simulink model "SmartHomeModelFinal"  (R2014a)
settings: Solver=ode45  StartTime=0.0  StopTime=inf  RelTol=1e-3
settings Model: Creator=Drazenko  LastModifiedBy=Drazenko

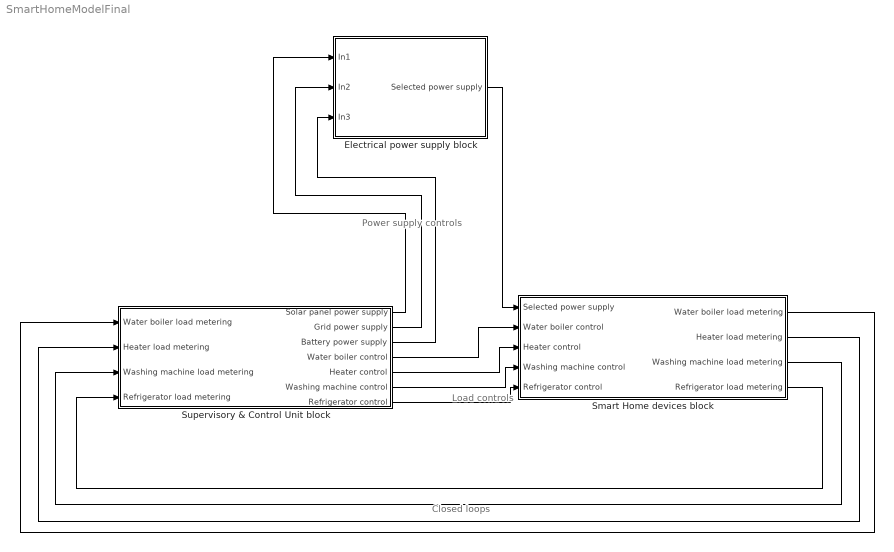
== system SmartHomeModelFinal ==
  note: Closed loops
  note: Load controls
  note: Power supply controls
  Electrical power supply block : Subsystem
  Smart Home devices block : Subsystem
  Supervisory & Control Unit block : Subsystem
  wires:
  Electrical power supply block/1(Selected power supply) -> Smart Home devices block/1(Selected power supply)
  Smart Home devices block/1(Water boiler load metering) -> Supervisory & Control Unit block/1(Water boiler load metering)
  Smart Home devices block/2(Heater load metering) -> Supervisory & Control Unit block/2(Heater load metering)
  Smart Home devices block/3(Washing machine load metering) -> Supervisory & Control Unit block/3(Washing machine load metering)
  Smart Home devices block/4(Refrigerator load metering) -> Supervisory & Control Unit block/4(Refrigerator load metering)
  Supervisory & Control Unit block/1(Solar panel power supply) -> Electrical power supply block/1(In1)
  Supervisory & Control Unit block/2(Grid power supply) -> Electrical power supply block/2(In2)
  Supervisory & Control Unit block/3(Battery power supply) -> Electrical power supply block/3(In3)
  Supervisory & Control Unit block/4(Water boiler control) -> Smart Home devices block/2(Water boiler control)
  Supervisory & Control Unit block/5(Heater control) -> Smart Home devices block/3(Heater control)
  Supervisory & Control Unit block/6(Washing machine control) -> Smart Home devices block/4(Washing machine control)
  Supervisory & Control Unit block/7(Refrigerator control) -> Smart Home devices block/5(Refrigerator control)

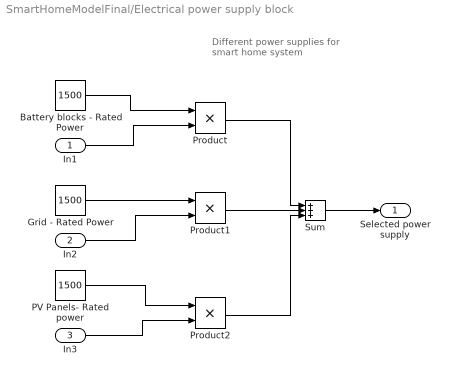
== system SmartHomeModelFinal/Electrical power supply block ==
  note: Different power supplies
      | for smart home system
  In1 : Inport
  In2 : Inport  Port=2
  In3 : Inport  Port=3
  Battery blocks - Rated Power : Constant  Value=1500
  Grid - Rated Power : Constant  Value=1500
  PV Panels- Rated power : Constant  Value=1500
  Product : Product
  Product1 : Product
  Product2 : Product
  Sum : Sum  Inputs=+++
  Selected power supply : Outport
  wires:
  Battery blocks - Rated Power/1 -> Product/1
  In1/1 -> Product/2
  Grid - Rated Power/1 -> Product1/1
  In2/1 -> Product1/2
  PV Panels- Rated power/1 -> Product2/1
  In3/1 -> Product2/2
  Product/1 -> Sum/1
  Product1/1 -> Sum/2
  Product2/1 -> Sum/3
  Sum/1 -> Selected power supply/1

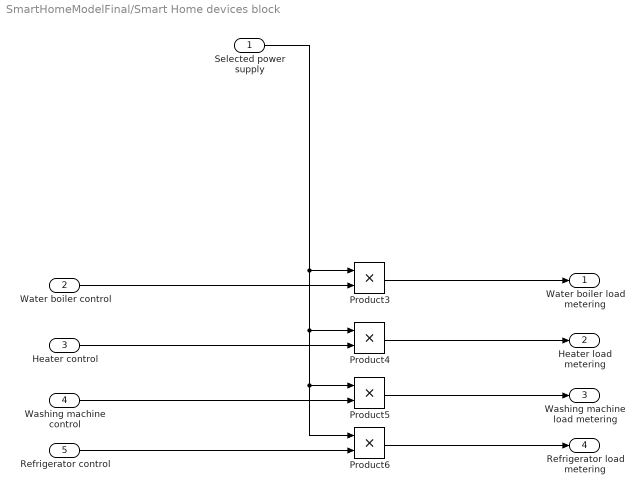
== system SmartHomeModelFinal/Smart Home devices block ==
  Selected power supply : Inport
  Water boiler control : Inport  Port=2
  Heater control : Inport  Port=3
  Washing machine control : Inport  Port=4
  Refrigerator control : Inport  Port=5
  Product{3..6} (4 alike) : Product
  Water boiler load metering : Outport
  Heater load metering : Outport  Port=2
  Washing machine load metering : Outport  Port=3
  Refrigerator load metering : Outport  Port=4
  wires:
  Water boiler control/1 -> Product3/2
  Selected power supply/1 -> Product6/1, Product5/1, Product4/1, Product3/1
  Heater control/1 -> Product4/2
  Washing machine control/1 -> Product5/2
  Refrigerator control/1 -> Product6/2
  Product3/1 -> Water boiler load metering/1
  Product4/1 -> Heater load metering/1
  Product5/1 -> Washing machine load metering/1
  Product6/1 -> Refrigerator load metering/1

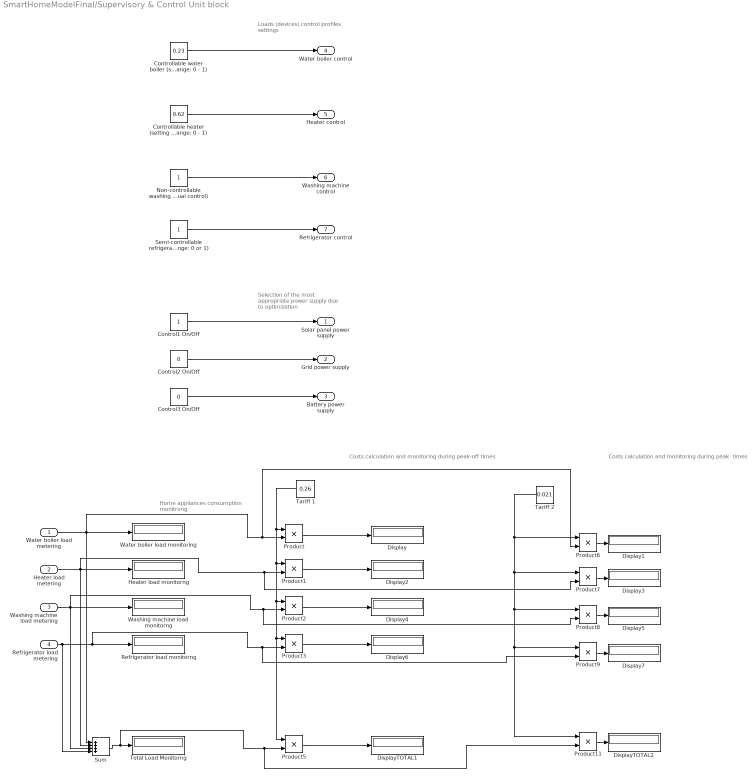
== system SmartHomeModelFinal/Supervisory & Control Unit block ==
  note: Loads (devices) control profiles
      | settings
  note: Home appliances consumption
      | monitrong
  note: Costs calculation and monitoring during peak- times
  note: Selection of the most
      | appropriate power supply
      | due to optimization
  note: Costs calculation and monitoring during peak-off times
  Water boiler load metering : Inport
  Heater load metering : Inport  Port=2
  Washing machine load metering : Inport  Port=3
  Refrigerator load metering : Inport  Port=4
  Control1 On/Off : Constant
  Control2 On/Off : Constant  Value=0
  Control3 On/Off : Constant  Value=0
  "Controllable water boiler (setting control parameter range: 0 - 1) " : Constant  Value=0.23
  Controllable heater (setting control parameter range: 0 - 1) : Constant  Value=0.62
  Display{,1..7} (8 alike) : Display
  DisplayTOTAL1 : Display
  DisplayTOTAL2 : Display
  Heater load monitorng : Display
  Non-controllable washing machine (depending on the manual control) : Constant
  Product{,1..3,5..9,11} (10 alike) : Product
  Refrigerator load monitorng : Display
  Semi-controllable refrigerator (setting control parameter range: 0 or 1) : Constant
  Sum : Sum  Inputs=++++
  Tariff 1 : Constant  Value=0.26
  Tariff 2 : Constant  Value=0.021
  Total Load Monitorng : Display
  Washing machine load monitorng : Display
  Water boiler load monitoring : Display
  Solar panel power supply : Outport
  Grid power supply : Outport  Port=2
  Battery power supply : Outport  Port=3
  Water boiler control : Outport  Port=4
  Heater control : Outport  Port=5
  Washing machine control : Outport  Port=6
  Refrigerator control : Outport  Port=7
  wires:
  "Controllable water boiler (setting control parameter range: 0 - 1) "/1 -> Water boiler control/1
  Controllable heater (setting control parameter range: 0 - 1)/1 -> Heater control/1
  Non-controllable washing machine (depending on the manual control)/1 -> Washing machine control/1
  Semi-controllable refrigerator (setting control parameter range: 0 or 1)/1 -> Refrigerator control/1
  Control1 On/Off/1 -> Solar panel power supply/1
  Control3 On/Off/1 -> Battery power supply/1
  Control2 On/Off/1 -> Grid power supply/1
  Water boiler load metering/1 -> Water boiler load monitoring/1, Sum/1, Product6/2, Product/2
  Heater load metering/1 -> Heater load monitorng/1, Product7/2, Product1/2, Sum/2
  Washing machine load metering/1 -> Washing machine load monitorng/1, Product8/2, Product2/2, Sum/3
  Refrigerator load metering/1 -> Product9/2, Product3/2, Refrigerator load monitorng/1, Sum/4
  Sum/1 -> Product11/2, Product5/2, Total Load Monitorng/1
  Tariff 1/1 -> Product5/1, Product3/1, Product2/1, Product1/1, Product/1
  Tariff 2/1 -> Product11/1, Product9/1, Product8/1, Product7/1, Product6/1
  Product/1 -> Display/1
  Product6/1 -> Display1/1
  Product7/1 -> Display3/1
  Product1/1 -> Display2/1
  Product2/1 -> Display4/1
  Product8/1 -> Display5/1
  Product3/1 -> Display6/1
  Product9/1 -> Display7/1
  Product11/1 -> DisplayTOTAL2/1
  Product5/1 -> DisplayTOTAL1/1
